simulink model "udp_testing"  (R2025b)
settings: Solver=VariableStepAuto  StartTime=0.0  StopTime=10.0  RelTol=1e-3
undefined symbols (not defined in the file or in its folder): f
libraries: instrumentlib x1
settings Model: Creator=sig  LastModifiedBy=sig

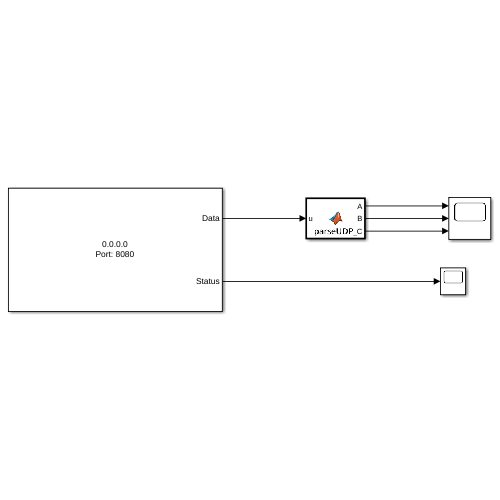
[thumbnail: Simulink's stored preview of the top-level diagram]
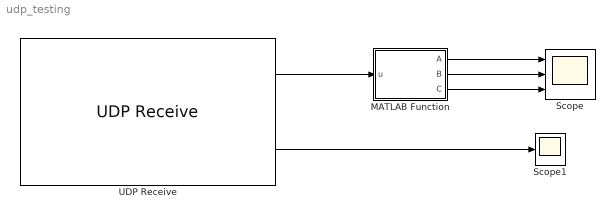
== system udp_testing ==
  MATLAB Function : MATLAB Function  TreatAsAtomicUnit=on
  Scope : Scope  NumInputPorts=3
      settings: ActiveDisplayYMinimum=-3.41425  ActiveDisplayYMaximum=3.62825
  Scope1 : Scope
      settings: ActiveDisplayYMinimum=-0.12499999999999997  ActiveDisplayYMaximum=1.125
  UDP Receive : instrumentlib/UDP Receive  LocalAddress=0.0.0.0  LocalPort=8080  EnablePortSharing=off  Host=localhost  Port=9090  GetLatestData=on  DataSize=[ 22, 1 ]  DataType=uint8  ASCIIFormatting=%f,  Terminator=LF  CustomTerminator=10  ByteOrder=big-endian  EnableBlockingMode=off  Timeout=10  SampleTime=0.01  SimulateUsing=Interpreted execution
  wires:
  UDP Receive/1 -> MATLAB Function/1(u)
  UDP Receive/2 -> Scope1/1
  MATLAB Function/1(A) -> Scope/1
  MATLAB Function/2(B) -> Scope/2
  MATLAB Function/3(C) -> Scope/3

== matlab function udp_testing/MATLAB Function ==
  data: u input; A output; B output; C output
function [A, B, C] = parseUDP_(u)

display(u)

A = 0.0; B = 0.0; C = 0.0;

u = char(u);
n = length(u);

currentAngle = '';
buffer = '';
newData = false;

for i = 1:n
    c = u(i);
    display(c)
    buffer = [buffer, c];
    switch c
        case 'A'
            currentAngle = 'A';
            newData = true;
        case 'B'
            currentAngle = 'B';
            newData = true;
        case 'C'
            currentAngle = 'C';
            newData = true;
        otherwise
            newData = false;
    end
    
    if ~isempty(currentAngle) && (buffer(1) ~= currentAngle(1)) && newData
        switch buffer(1)
            case 'A'
                A = real(str2double(buffer(3:end-1)));
            case 'B'
                B = real(str2double(buffer(3:end-1)));
            case 'C'
                C = real(str2double(buffer(3:end-1)));
        end
    buffer = currentAngle;
    end
end
switch currentAngle
    case 'A'
        A = real(str2double(buffer(3:end-1)));
    case 'B'
        B = real(str2double(buffer(3:end-1)));
    case 'C'
        C = real(str2double(buffer(3:end-1)));
end
